simulink model "PID_Pendulum_ROS"  (R2020b)
settings: Solver=ode4  StartTime=0.0  StopTime=10  FixedStep=1e-3  RelTol=1e-3
libraries: robotlib x4
settings Model: Creator=gabriel  LastModifiedBy=gabriel

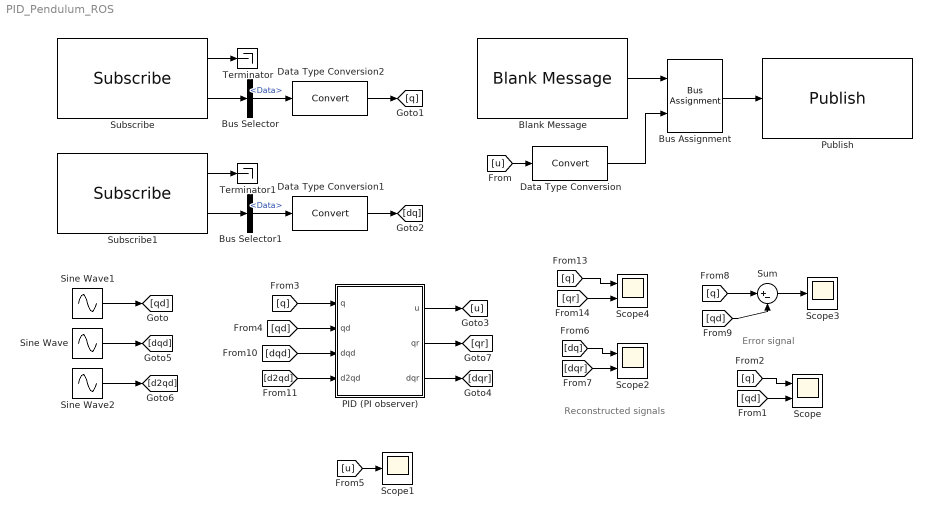
== system PID_Pendulum_ROS ==
  note: Error signal
  note: Reconstructed signals
  Blank Message : robotlib/Blank Message  messageClass=Message  entityType=std_msgs/Float32  messageType=std_msgs/Float32  SampleTime=inf  legacyBusStruct=off
  Bus Assignment : BusAssignment  AssignedSignals=Data
  Bus Selector : BusSelector  OutputSignals=Data
  Bus Selector1 : BusSelector  OutputSignals=Data
  Data Type Conversion : DataTypeConversion
  Data Type Conversion1 : DataTypeConversion
  Data Type Conversion2 : DataTypeConversion
  PID (PI observer) : Subsystem  mask{m=0.3125, l=0.5, k2=50, k1=5000, k0=50}
      mask prompts: m "Mass"; l "Length"
      mask init:
      | g = 9.81;
      | J = 1/3*m*l^2;
      | Jmassless = J/m;
  Publish : robotlib/Publish  topicSource=Specify your own  topic=/u  messageType=std_msgs/Float32  legacyBusStruct=off  messageQueueLength=1
  Scope : Scope  NumInputPorts=2
  Scope1 : Scope
  Scope2 : Scope  NumInputPorts=2
  Scope3 : Scope
  Scope4 : Scope  NumInputPorts=2
  Sine Wave : Sin  Amplitude=1.5  Phase=pi/2  SampleTime=0
  Sine Wave1 : Sin  Amplitude=1.5  SampleTime=0
  Sine Wave2 : Sin  Amplitude=1.5  Phase=-pi  SampleTime=0
  Subscribe : robotlib/Subscribe  topicSource=Select from ROS network  topic=/q  messageType=std_msgs/Float32  SampleTime=-1  legacyBusStruct=off  messageQueueLength=1
  Subscribe1 : robotlib/Subscribe  topicSource=Select from ROS network  topic=/dq  messageType=std_msgs/Float32  SampleTime=-1  legacyBusStruct=off  messageQueueLength=1
  Sum : Sum  Inputs=|+-
  Terminator : Terminator
  Terminator1 : Terminator
  wires:
  Sine Wave/1 -> [dqd]
  [q] -> Scope/1
  [u] -> Scope1/1
  [qd] -> Sum/2
  Sine Wave2/1 -> [d2qd]
  PID (PI observer)/1(u) -> [u]
  [q] -> PID (PI observer)/1(q)
  [qd] -> Scope/2
  [d2qd] -> PID (PI observer)/4(d2qd)
  Sine Wave1/1 -> [qd]
  [dqd] -> PID (PI observer)/3(dqd)
  [q] -> Sum/1
  [qd] -> PID (PI observer)/2(qd)
  PID (PI observer)/3(dqr) -> [dqr]
  Sum/1 -> Scope3/1
  Subscribe/1 -> Terminator/1
  Blank Message/1 -> Bus Assignment/1
  Bus Assignment/1 -> Publish/1
  Data Type Conversion/1 -> Bus Assignment/2
  [u] -> Data Type Conversion/1
  Subscribe1/1 -> Terminator1/1
  Subscribe/2 -> Bus Selector/1
  Subscribe1/2 -> Bus Selector1/1
  Data Type Conversion1/1 -> [dq]
  Bus Selector1/1 -> Data Type Conversion1/1  "<Data>"
  Bus Selector/1 -> Data Type Conversion2/1  "<Data>"
  Data Type Conversion2/1 -> [q]
  PID (PI observer)/2(qr) -> [qr]
  [q] -> Scope4/1
  [qr] -> Scope4/2
  [dq] -> Scope2/1
  [dqr] -> Scope2/2

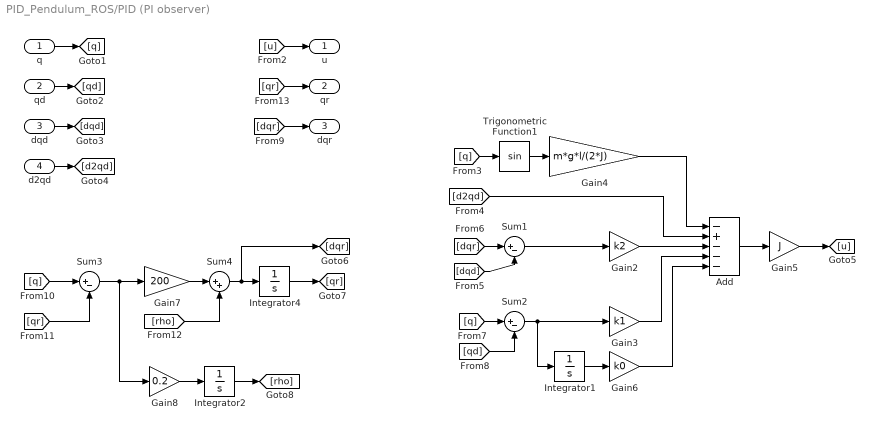
== system PID_Pendulum_ROS/PID (PI observer) ==
  q : Inport
  qd : Inport  Port=2
  dqd : Inport  Port=3
  d2qd : Inport  Port=4
  Add : Sum  Inputs=-+---
  Gain2 : Gain  Gain=k2
  Gain3 : Gain  Gain=k1
  Gain4 : Gain  Gain=m*g*l/(2*J)
  Gain5 : Gain  Gain=J
  Gain6 : Gain  Gain=k0
  Gain7 : Gain  Gain=200
  Gain8 : Gain  Gain=0.2
  Integrator1 : Integrator
  Integrator2 : Integrator
  Integrator4 : Integrator
  Sum1 : Sum  Inputs=|+-
  Sum2 : Sum  Inputs=|+-
  Sum3 : Sum  Inputs=|+-
  Sum4 : Sum  Inputs=|++
  Trigonometric Function1 : Trigonometry
  u : Outport
  qr : Outport  Port=2
  dqr : Outport  Port=3
  wires:
  q/1 -> [q]
  qd/1 -> [qd]
  dqd/1 -> [dqd]
  [u] -> u/1
  [q] -> Trigonometric Function1/1
  d2qd/1 -> [d2qd]
  [dqr] -> Sum1/1
  [dqd] -> Sum1/2
  Sum1/1 -> Gain2/1
  [q] -> Sum2/1
  [qd] -> Sum2/2
  Sum2/1 -> Integrator1/1, Gain3/1
  Gain2/1 -> Add/3
  Gain3/1 -> Add/4
  [d2qd] -> Add/2
  Trigonometric Function1/1 -> Gain4/1
  Gain4/1 -> Add/1
  Add/1 -> Gain5/1
  Gain5/1 -> [u]
  Integrator1/1 -> Gain6/1
  Gain6/1 -> Add/5
  [dqr] -> dqr/1
  [q] -> Sum3/1
  [qr] -> Sum3/2
  Sum3/1 -> Gain8/1, Gain7/1
  Gain7/1 -> Sum4/1
  [rho] -> Sum4/2
  Gain8/1 -> Integrator2/1
  Sum4/1 -> [dqr], Integrator4/1
  Integrator4/1 -> [qr]
  Integrator2/1 -> [rho]
  [qr] -> qr/1
